simulink model "simpleStateflowModel"  (R2020b)
settings: Solver=VariableStepAuto  StartTime=0.0  StopTime=10.0  RelTol=1e-3
settings Model: Creator=aarrieta  LastModifiedBy=aarrieta

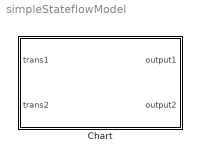
== system simpleStateflowModel ==
  Chart : Stateflow chart  TreatAsAtomicUnit=on

== stateflow chart simpleStateflowModel/Chart ==
  state State2
    during:
    output2 = 2-11/3-13+6;
    output1=0*16;
  state State1
    entry:
    output1 =1;
    entry:
    output1 = 2;
  state State3
    entry:
    output1 = 3;
  (default) -> State2
  State1 -> State2 : [trans1<5 && trans2 == 5 ||after(5,sec)]
  State2 -> State3 : [trans2== 5 && trans1 < 3]
  State3 -> State2 [order 1] : [trans2 <0 && trans1<5]
  State3 -> State1 [order 2] : [after(5,msec)&&trans1 ==3]
  data: trans1 input; trans2 input; output1 output; output2 output
